simulink model "qmult_test2"  (Simulink 7.0)
settings: Solver=FixedStepDiscrete  StartTime=0.0  StopTime=stop_time  FixedStep=1.0  RelTol=1e-3
libraries: simulink x4
Description:
  | Timing Test: Quaternion Multiplication, method 2
  | 
  | Copyright (c) 2001-2009, Jay A. St. Pierre.  All rights reserved.
settings Model: Creator=stpierre  LastModifiedBy=stpierre  ExtModeTrigMode=oneshot  ExtModeArmWhenConnect=off  ExtModeAutoUpdateStatusClock=off
settings DataIOCC: MaxDataPoints=1  SaveOutput=off  SaveTime=off
settings OptimizationCC: BlockReduction=off  BooleanDataType=off
settings DebuggingCC: SaveWithParameterizedLinksMsg=none  SignalResolutionControl=TryResolveAllWithWarning  SolverPrmCheckMsg=none  MultiTaskDSMMsg=warning  MultiTaskCondExecSysMsg=none  StrictBusMsg=None
settings HardwareCC: TargetUnknown=on
settings RTWCC: IncludeERTFirstTime=on

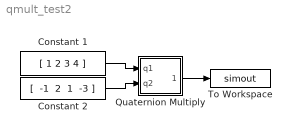
== system qmult_test2 ==
  Constant 1 : Constant  Value=[ 1 2 3 4 ]
  Constant 2 : Constant  Value="[  -1  2  1  -3 ]"
  Quaternion Multiply : Subsystem
      mask Type: Quaternion Multiply
      mask Description: q3 = (q1)(q2)
  To Workspace : ToWorkspace  VariableName=simout  SampleTime=-1  SaveFormat=Array
      settings: MaxDataPoints=1
  wires:
  Constant 1/1 -> Quaternion Multiply/1(q1)
  Quaternion Multiply/1(q1q2) -> To Workspace/1
  Constant 2/1 -> Quaternion Multiply/2(q2)

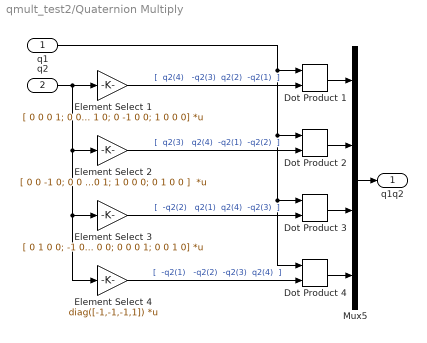
== system qmult_test2/Quaternion Multiply ==
  q1 : Inport  PortDimensions=4
  q2 : Inport  Port=2  PortDimensions=4
  Dot Product {1..4} (4 alike) : simulink/Math Operations/Dot Product  InputSameDT=on  OutDataType=sfix(16)  OutScaling=2^-10  DoSatur=off
  Element Select 1 : Gain  Gain=[ 0 0 0 1; 0 0 1 0; 0 -1 0 0; 1 0 0 0]  Multiplication=Matrix(K*u)  ParameterDataType=sfix(16)  ParameterScaling=2^0  OutDataType=sfix(16)  OutScaling=2^0  SaturateOnIntegerOverflow=on
  Element Select 2 : Gain  Gain=[ 0 0 -1 0; 0 0 0 1; 1 0 0 0; 0 1 0 0 ]  Multiplication=Matrix(K*u)  ParameterDataType=sfix(16)  ParameterScaling=2^0  OutDataType=sfix(16)  OutScaling=2^0  SaturateOnIntegerOverflow=on
  Element Select 3 : Gain  Gain=[ 0 1 0 0; -1 0 0 0; 0 0 0 1; 0 0 1 0]  Multiplication=Matrix(K*u)  ParameterDataType=sfix(16)  ParameterScaling=2^0  OutDataType=sfix(16)  OutScaling=2^0  SaturateOnIntegerOverflow=on
  Element Select 4 : Gain  Gain=diag([-1,-1,-1,1])  Multiplication=Matrix(K*u)  ParameterDataType=sfix(16)  ParameterScaling=2^0  OutDataType=sfix(16)  OutScaling=2^0  SaturateOnIntegerOverflow=on
  Mux5 : Mux
  q1q2 : Outport  InitialOutput=0
  wires:
  q2/1 -> Element Select 1/1, Element Select 2/1, Element Select 3/1, Element Select 4/1
  Dot Product 2/1 -> Mux5/2
  Dot Product 1/1 -> Mux5/1
  q1/1 -> Dot Product 4/1, Dot Product 3/1, Dot Product 2/1, Dot Product 1/1
  Element Select 1/1 -> Dot Product 1/2  "[  q2(4)   -q2(3)  q2(2)  -q2(1)  ]"
  Mux5/1 -> q1q2/1
  Element Select 2/1 -> Dot Product 2/2  "[  q2(3)   q2(4)  -q2(1)  -q2(2)  ]"
  Dot Product 3/1 -> Mux5/3
  Element Select 3/1 -> Dot Product 3/2  "[  -q2(2)   q2(1)  q2(4)  -q2(3)  ]"
  Dot Product 4/1 -> Mux5/4
  Element Select 4/1 -> Dot Product 4/2  "[  -q2(1)   -q2(2)  -q2(3)  q2(4)  ]"
